simulink model "torqueBalancingPHRIStandup"  (Simulink 9.1)
settings: Solver=FixedStepDiscrete  StartTime=0.0  StopTime="Config.SIMULATION_TIME "  FixedStep=Config.Ts  RelTol=1e-3  EnableMultiTasking=on
StopFcn:
  | cd(fileparts(which(bdroot)));
  | stopTorqueBalancingPHRIStandup;
undefined symbols (not defined in the file or in its folder): ASSISTANT_DOF_FOR_SIMULINK, bVectorConstraintsFeet, bVectorConstraintsLegs, Config, ConstraintsMatrixFeet, ConstraintsMatrixLegs, Gain, Reg, ROBOT_DOF, ROBOT_DOF_FOR_SIMULINK, Sat, Sm
libraries: WBToolboxLibrary x154, simulink x4
(part 1 of 4)
settings Model: SuppressorTable=22 serialization::archive 11 0 6 0 0 0 1 0  Creator=daniele  LastModifiedBy=yeshi  NumberOfSteps=100
settings DataIOCC: LimitDataPoints=on
settings OptimizationCC: ExpressionDepthLimit=2147483647
settings DebuggingCC: SolverPrmCheckMsg=warning  FcnCallInpInsideContextMsg=warning  AllowSymbolicDim=off  StateNameClashWarn=warning
settings SFSimCC: SimParseCustomCode=off
settings GRTTargetCC: GeneratePreprocessorConditionals=Disable all

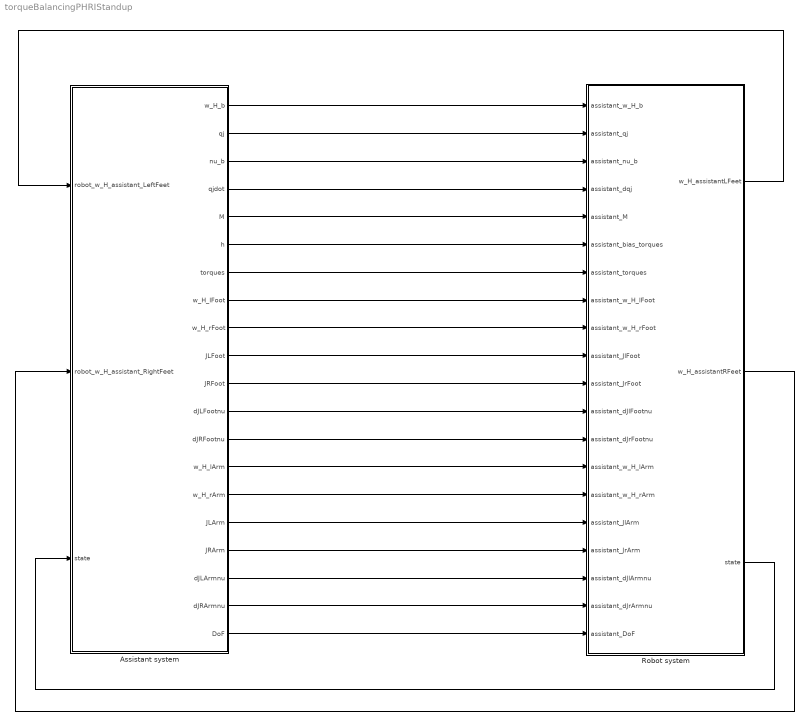
== system torqueBalancingPHRIStandup ==
  Assistant system : Subsystem
  Robot system : Subsystem
  wires:
  Assistant system/1(w_H_b) -> Robot system/1("assistant_w_H_b ")
  Assistant system/2(qj) -> Robot system/2("assistant_qj ")
  Assistant system/3(nu_b) -> Robot system/3(assistant_nu_b)
  Assistant system/4(qjdot) -> Robot system/4(assistant_dqj)
  Assistant system/5(M) -> Robot system/5(assistant_M)
  Assistant system/6(h) -> Robot system/6(assistant_bias_torques)
  Assistant system/7(torques) -> Robot system/7(assistant_torques)
  Assistant system/8(w_H_lFoot) -> Robot system/8(assistant_w_H_lFoot)
  Assistant system/9(w_H_rFoot) -> Robot system/9(assistant_w_H_rFoot)
  Assistant system/10(JLFoot) -> Robot system/10(assistant_JlFoot)
  Assistant system/11(JRFoot) -> Robot system/11(assistant_JrFoot)
  Assistant system/12(dJLFootnu) -> Robot system/12(assistant_dJlFootnu)
  Assistant system/13(dJRFootnu) -> Robot system/13(assistant_dJrFootnu)
  Assistant system/14(w_H_lArm) -> Robot system/14(assistant_w_H_lArm)
  Assistant system/15(w_H_rArm) -> Robot system/15(assistant_w_H_rArm)
  Assistant system/16(JLArm) -> Robot system/16(assistant_JlArm)
  Assistant system/17(JRArm) -> Robot system/17(assistant_JrArm)
  Assistant system/18(dJLArmnu) -> Robot system/18(assistant_dJlArmnu)
  Assistant system/19(dJRArmnu) -> Robot system/19(assistant_dJrArmnu)
  Assistant system/20(DoF) -> Robot system/20(assistant_DoF)
  Robot system/1(w_H_assistantLFeet) -> Assistant system/1(robot_w_H_assistant_LeftFeet)
  Robot system/2(w_H_assistantRFeet) -> Assistant system/2(robot_w_H_assistant_RightFeet)
  Robot system/3(state) -> Assistant system/3("state ")

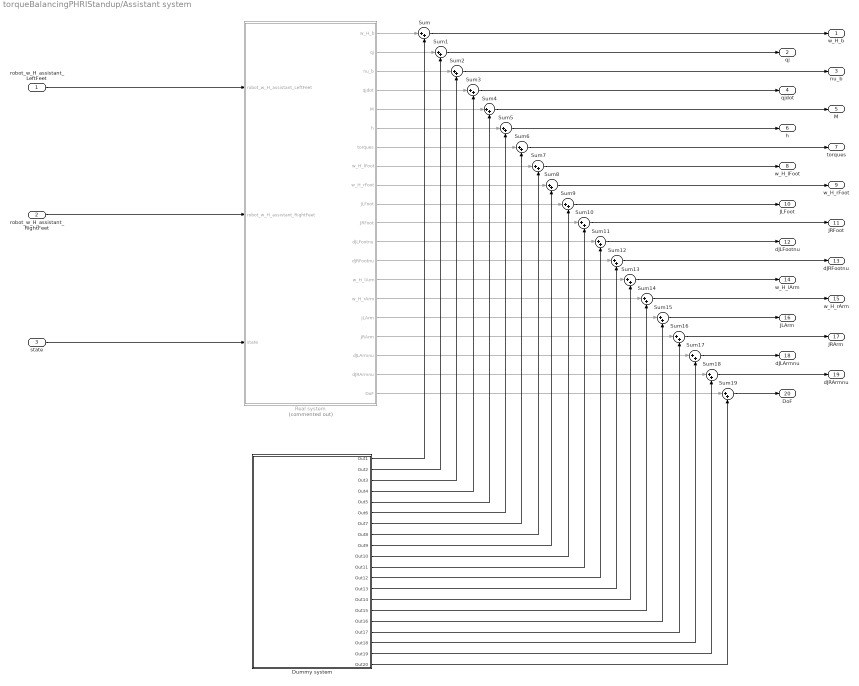
== system torqueBalancingPHRIStandup/Assistant system ==
  robot_w_H_assistant_LeftFeet : Inport
  robot_w_H_assistant_RightFeet : Inport  Port=2
  "state " : Inport  Port=3
  Dummy system : Subsystem
  Real system : Subsystem  Commented=on
  Sum{,1..19} (20 alike) : Sum  Inputs=|++
  w_H_b : Outport
  qj : Outport  Port=2
  nu_b : Outport  Port=3
  qjdot : Outport  Port=4
  M : Outport  Port=5
  h : Outport  Port=6
  torques : Outport  Port=7
  w_H_lFoot : Outport  Port=8
  w_H_rFoot : Outport  Port=9
  JLFoot : Outport  Port=10
  JRFoot : Outport  Port=11
  dJLFootnu : Outport  Port=12
  dJRFootnu : Outport  Port=13
  w_H_lArm : Outport  Port=14
  w_H_rArm : Outport  Port=15
  JLArm : Outport  Port=16
  JRArm : Outport  Port=17
  dJLArmnu : Outport  Port=18
  dJRArmnu : Outport  Port=19
  DoF : Outport  Port=20
  wires:
  robot_w_H_assistant_LeftFeet/1 -> Real system/1(robot_w_H_assistant_LeftFeet)
  robot_w_H_assistant_RightFeet/1 -> Real system/2(robot_w_H_assistant_RightFeet)
  "state "/1 -> Real system/3("state ")
  Sum/1 -> w_H_b/1
  Real system/1(w_H_b) -> Sum/1
  Real system/2(qj) -> Sum1/1
  Sum1/1 -> qj/1
  Real system/3(nu_b) -> Sum2/1
  Sum2/1 -> nu_b/1
  Real system/4(qjdot) -> Sum3/1
  Sum3/1 -> qjdot/1
  Real system/5(M) -> Sum4/1
  Sum4/1 -> M/1
  Real system/6(h) -> Sum5/1
  Sum5/1 -> h/1
  Real system/7(torques) -> Sum6/1
  Sum6/1 -> torques/1
  Real system/8(w_H_lFoot) -> Sum7/1
  Sum7/1 -> w_H_lFoot/1
  Real system/9(w_H_rFoot) -> Sum8/1
  Sum8/1 -> w_H_rFoot/1
  Real system/10(JLFoot) -> Sum9/1
  Sum9/1 -> JLFoot/1
  Real system/11(JRFoot) -> Sum10/1
  Sum10/1 -> JRFoot/1
  Real system/12(dJLFootnu) -> Sum11/1
  Sum11/1 -> dJLFootnu/1
  Real system/13(dJRFootnu) -> Sum12/1
  Sum12/1 -> dJRFootnu/1
  Real system/14(w_H_lArm) -> Sum13/1
  Sum13/1 -> w_H_lArm/1
  Real system/15(w_H_rArm) -> Sum14/1
  Sum14/1 -> w_H_rArm/1
  Real system/16(JLArm) -> Sum15/1
  Sum15/1 -> JLArm/1
  Real system/17(JRArm) -> Sum16/1
  Sum16/1 -> JRArm/1
  Real system/18(dJLArmnu) -> Sum17/1
  Sum17/1 -> dJLArmnu/1
  Real system/19(dJRArmnu) -> Sum18/1
  Sum18/1 -> dJRArmnu/1
  Sum19/1 -> DoF/1
  Real system/20(DoF) -> Sum19/1
  Dummy system/1(Out1) -> Sum/2
  Dummy system/2(Out2) -> Sum1/2
  Dummy system/3(Out3) -> Sum2/2
  Dummy system/4(Out4) -> Sum3/2
  Dummy system/5(Out5) -> Sum4/2
  Dummy system/6(Out6) -> Sum5/2
  Dummy system/7(Out7) -> Sum6/2
  Dummy system/8(Out8) -> Sum7/2
  Dummy system/9(Out9) -> Sum8/2
  Dummy system/10(Out10) -> Sum9/2
  Dummy system/11(Out11) -> Sum10/2
  Dummy system/12(Out12) -> Sum11/2
  Dummy system/13(Out13) -> Sum12/2
  Dummy system/14(Out14) -> Sum13/2
  Dummy system/15(Out15) -> Sum14/2
  Dummy system/16(Out16) -> Sum15/2
  Dummy system/17(Out17) -> Sum16/2
  Dummy system/18(Out18) -> Sum17/2
  Dummy system/19(Out19) -> Sum18/2
  Dummy system/20(Out20) -> Sum19/2

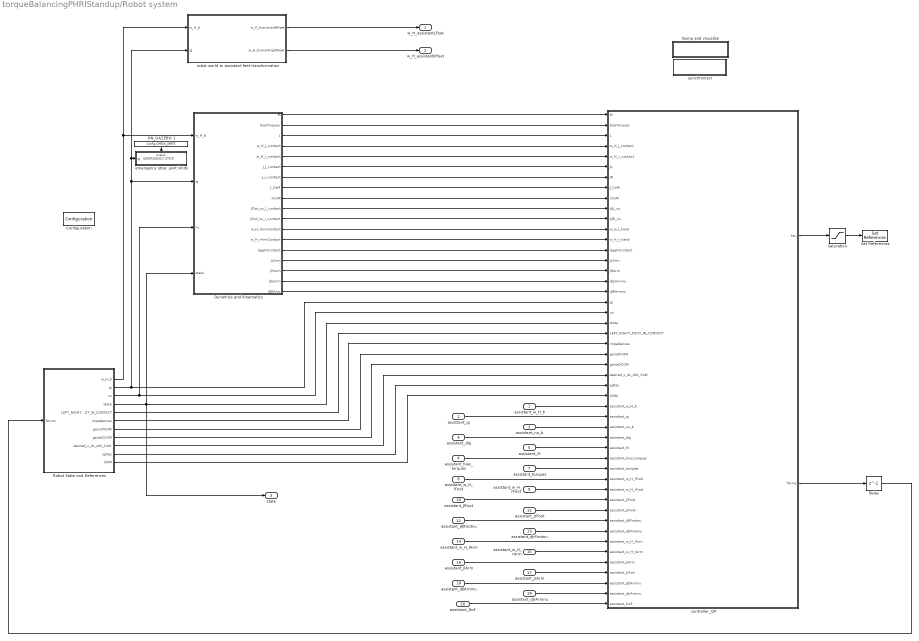
== system torqueBalancingPHRIStandup/Robot system ==
  "assistant_w_H_b " : Inport
  "assistant_qj " : Inport  Port=2
  assistant_nu_b : Inport  Port=3
  assistant_dqj : Inport  Port=4
  assistant_M : Inport  Port=5
  assistant_bias_torques : Inport  Port=6
  assistant_torques : Inport  Port=7
  assistant_w_H_lFoot : Inport  Port=8
  assistant_w_H_rFoot : Inport  Port=9
  assistant_JlFoot : Inport  Port=10
  assistant_JrFoot : Inport  Port=11
  assistant_dJlFootnu : Inport  Port=12
  assistant_dJrFootnu : Inport  Port=13
  assistant_w_H_lArm : Inport  Port=14
  assistant_w_H_rArm : Inport  Port=15
  assistant_JlArm : Inport  Port=16
  assistant_JrArm : Inport  Port=17
  assistant_dJlArmnu : Inport  Port=18
  assistant_dJrArmnu : Inport  Port=19
  assistant_DoF : Inport  Port=20
  Configuration : WBToolboxLibrary/Utilities/Configuration  ConfigSource=Workspace  ConfigObject='WBTConfigRobot'
      settings: SourceProductName=Whole Body Toolbox
  Delay : Delay  DelayLength=1
  Dump and visualize : Subsystem
      mask Display: disp('VISUALIZER')
  Dynamics and Kinematics : Subsystem
  ON_GAZEBO 1 : Constant  Value=Config.CHECK_LIMITS
  Robot State and References : Subsystem  Priority=-10
  Saturation : Saturate  UpperLimit=Sat.torque  LowerLimit=-Sat.torque
  Set References : WBToolboxLibrary/wholeBodyActuators/Set References  controlType=Torque  refSpeed=50  refAcceleration=1000000*(pi/180)
      settings: SourceProductName=Whole Body Toolbox
  controller_QP : Subsystem
  emergency stop: joint limits : Subsystem
  robot world to assistant feet transformation : Subsystem
  synchronizer : Subsystem
      mask Display: disp('SYNCHRONIZER')
  w_H_assistantLFeet : Outport
  w_H_assistantRFeet : Outport  Port=2
  state : Outport  Port=3
  wires:
  Dynamics and Kinematics/9(xCoM) -> controller_QP/9(xCoM)
  Saturation/1 -> Set References/1
  Robot State and References/6(impedances) -> controller_QP/23(impedances)
  Robot State and References/7(gainsPCOM) -> controller_QP/24(gainsPCOM)
  Dynamics and Kinematics/10(JDot_nu_l_contact) -> controller_QP/10(dJL_nu)
  Robot State and References/5(LEFT_RIGHT_FOOT_IN_CONTACT) -> controller_QP/22(LEFT_RIGHT_FOOT_IN_CONTACT)
  Dynamics and Kinematics/2(biasTorques) -> controller_QP/2(biasTorques)
  ON_GAZEBO 1/1 -> emergency stop: joint limits/Enable
  Dynamics and Kinematics/6(J_l_contact) -> controller_QP/6(JL)
  Dynamics and Kinematics/14(legsInContact) -> controller_QP/14(legsInContact)
  Dynamics and Kinematics/8(J_CoM) -> controller_QP/8(J_CoM)
  Robot State and References/4(state) -> state/1, Dynamics and Kinematics/4("state "), controller_QP/21(state)
  Dynamics and Kinematics/4(w_H_l_contact) -> controller_QP/4(w_H_l_contact)
  Robot State and References/2(qj) -> robot world to assistant feet transformation/2(qj), emergency stop: joint limits/1(qj   EMERGENCY STOP), Dynamics and Kinematics/2(qj), controller_QP/19(qj)
  Dynamics and Kinematics/11(JDot_nu_r_contact) -> controller_QP/11(dJR_nu)
  Robot State and References/10(qjDes) -> controller_QP/27(qjDes)
  Robot State and References/9(desired_x_dx_ddx_CoM) -> controller_QP/26(desired_x_dx_ddx_CoM)
  Dynamics and Kinematics/1(M) -> controller_QP/1(M)
  Dynamics and Kinematics/5(w_H_r_contact) -> controller_QP/5(w_H_r_contact)
  Robot State and References/8(gainsDCOM) -> controller_QP/25(gainsDCOM)
  Robot State and References/1(w_H_b) -> robot world to assistant feet transformation/1(w_H_b), Dynamics and Kinematics/1(w_H_b)
  Robot State and References/3(nu) -> Dynamics and Kinematics/3(nu), controller_QP/20(nu)
  controller_QP/1("tau ") -> Saturation/1
  Dynamics and Kinematics/7(J_r_contact) -> controller_QP/7(JR)
  Dynamics and Kinematics/3(L) -> controller_QP/3("L ")
  robot world to assistant feet transformation/2(w_H_humanRightFeet) -> w_H_assistantRFeet/1
  robot world to assistant feet transformation/1(w_H_humanLeftFeet) -> w_H_assistantLFeet/1
  "assistant_w_H_b "/1 -> controller_QP/29("assistant_w_H_b ")
  "assistant_qj "/1 -> controller_QP/30("assistant_qj ")
  assistant_nu_b/1 -> controller_QP/31(assistant_nu_b)
  assistant_dqj/1 -> controller_QP/32(assistant_dqj)
  assistant_M/1 -> controller_QP/33(assistant_M)
  assistant_bias_torques/1 -> controller_QP/34(assistant_bias_torques)
  assistant_torques/1 -> controller_QP/35(assistant_torques)
  assistant_w_H_lFoot/1 -> controller_QP/36(assistant_w_H_lFoot)
  assistant_w_H_rFoot/1 -> controller_QP/37(assistant_w_H_rFoot)
  assistant_JlFoot/1 -> controller_QP/38(assistant_JlFoot)
  assistant_JrFoot/1 -> controller_QP/39(assistant_JrFoot)
  assistant_dJlFootnu/1 -> controller_QP/40(assistant_dJlFootnu)
  assistant_dJrFootnu/1 -> controller_QP/41(assistant_dJrFootnu)
  assistant_w_H_lArm/1 -> controller_QP/42(assistant_w_H_lArm)
  assistant_w_H_rArm/1 -> controller_QP/43(assistant_w_H_rArm)
  assistant_JlArm/1 -> controller_QP/44(assistant_JlArm)
  assistant_JrArm/1 -> controller_QP/45(assistant_JrArm)
  assistant_dJlArmnu/1 -> controller_QP/46(assistant_dJlArmnu)
  assistant_dJrArmnu/1 -> controller_QP/47(assistant_dJrArmnu)
  assistant_DoF/1 -> controller_QP/48(assistant_DoF)
  Dynamics and Kinematics/12(w_H_lArmContact) -> controller_QP/12(w_H_l_hand)
  Dynamics and Kinematics/13(w_H_rArmContact) -> controller_QP/13(w_H_r_hand)
  Dynamics and Kinematics/15(JLArm) -> controller_QP/15(JLArm)
  Dynamics and Kinematics/16(JRArm) -> controller_QP/16(JRArm)
  Dynamics and Kinematics/17(dJLArm) -> controller_QP/17(dJLArmnu)
  Dynamics and Kinematics/18(dJRArm) -> controller_QP/18(dJRArmnu)
  controller_QP/2(fArms) -> Delay/1
  Delay/1 -> Robot State and References/1(fArms)
  Robot State and References/11(CMM) -> controller_QP/28(CMM)

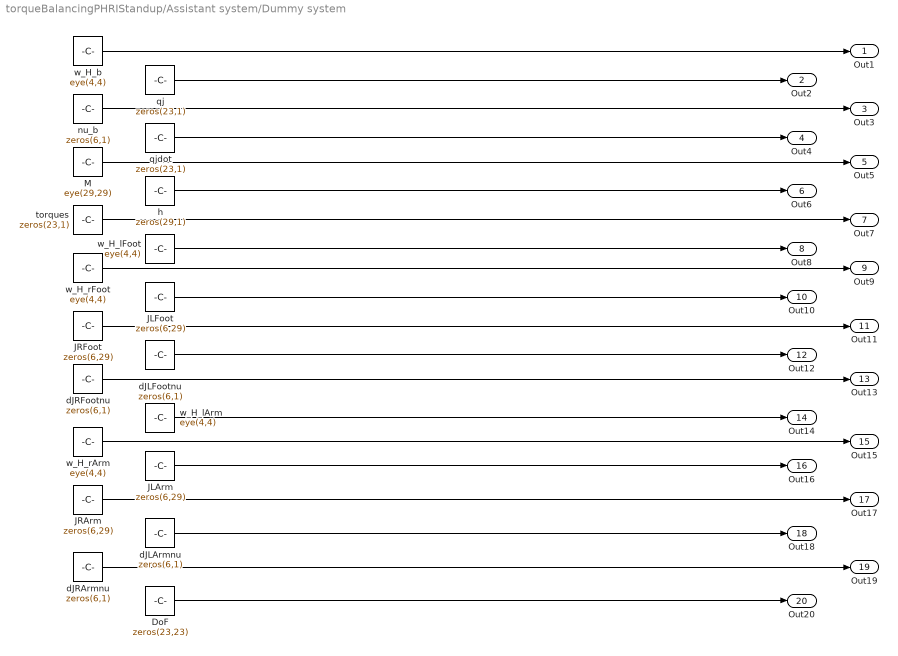
== system torqueBalancingPHRIStandup/Assistant system/Dummy system ==
  DoF : Constant  Value=zeros(23,23)
  JLArm : Constant  Value=zeros(6,29)
  "JLFoot " : Constant  Value=zeros(6,29)
  JRArm : Constant  Value=zeros(6,29)
  JRFoot : Constant  Value=zeros(6,29)
  M : Constant  Value=eye(29,29)
  dJLArmnu : Constant  Value=zeros(6,1)
  dJLFootnu : Constant  Value=zeros(6,1)
  dJRArmnu : Constant  Value=zeros(6,1)
  dJRFootnu : Constant  Value=zeros(6,1)
  "h " : Constant  Value=zeros(29,1)
  nu_b : Constant  Value=zeros(6,1)
  qj : Constant  Value=zeros(23,1)
  qjdot : Constant  Value=zeros(23,1)
  torques : Constant  Value=zeros(23,1)
  w_H_b : Constant  Value=eye(4,4)
  "w_H_lArm " : Constant  Value=eye(4,4)
  w_H_lFoot : Constant  Value=eye(4,4)
  "w_H_rArm " : Constant  Value=eye(4,4)
  "w_H_rFoot " : Constant  Value=eye(4,4)
  Out1 : Outport
  Out2 : Outport  Port=2
  Out3 : Outport  Port=3
  Out4 : Outport  Port=4
  Out5 : Outport  Port=5
  Out6 : Outport  Port=6
  Out7 : Outport  Port=7
  Out8 : Outport  Port=8
  Out9 : Outport  Port=9
  Out10 : Outport  Port=10
  Out11 : Outport  Port=11
  Out12 : Outport  Port=12
  Out13 : Outport  Port=13
  Out14 : Outport  Port=14
  Out15 : Outport  Port=15
  Out16 : Outport  Port=16
  Out17 : Outport  Port=17
  Out18 : Outport  Port=18
  Out19 : Outport  Port=19
  Out20 : Outport  Port=20
  wires:
  nu_b/1 -> Out3/1
  DoF/1 -> Out20/1
  JRArm/1 -> Out17/1
  "w_H_lArm "/1 -> Out14/1
  "w_H_rArm "/1 -> Out15/1
  dJRArmnu/1 -> Out19/1
  w_H_lFoot/1 -> Out8/1
  "JLFoot "/1 -> Out10/1
  torques/1 -> Out7/1
  qjdot/1 -> Out4/1
  w_H_b/1 -> Out1/1
  dJRFootnu/1 -> Out13/1
  dJLArmnu/1 -> Out18/1
  qj/1 -> Out2/1
  "h "/1 -> Out6/1
  dJLFootnu/1 -> Out12/1
  "w_H_rFoot "/1 -> Out9/1
  JRFoot/1 -> Out11/1
  JLArm/1 -> Out16/1
  M/1 -> Out5/1

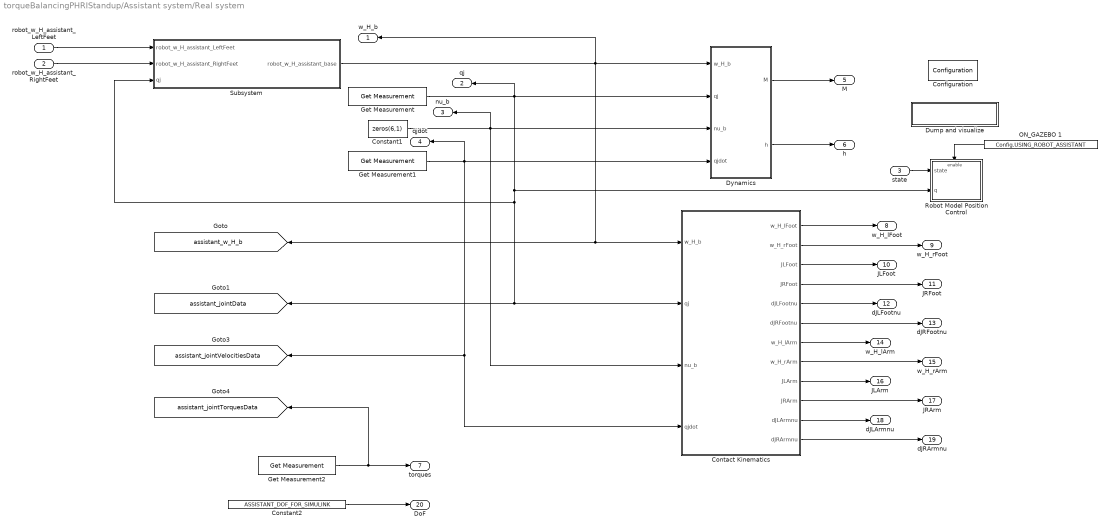
== system torqueBalancingPHRIStandup/Assistant system/Real system ==
  robot_w_H_assistant_LeftFeet : Inport
  robot_w_H_assistant_RightFeet : Inport  Port=2
  "state " : Inport  Port=3
  Configuration : WBToolboxLibrary/Utilities/Configuration  ConfigSource=Workspace  ConfigObject='ASSISTANT_WBTConfigRobot'
      settings: SourceProductName=Whole Body Toolbox
  Constant1 : Constant  Value=zeros(6,1)
  Constant2 : Constant  Value=ASSISTANT_DOF_FOR_SIMULINK
  Contact Kinematics : Subsystem
  Dump and visualize : Subsystem
      mask Display: disp('VISUALIZER')
  Dynamics : Subsystem
  Get Measurement : WBToolboxLibrary/wholeBodyStates/Get Measurement  measuredType=Joints Position
      settings: SourceProductName=Whole Body Toolbox
  Get Measurement1 : WBToolboxLibrary/wholeBodyStates/Get Measurement  measuredType=Joints Velocity
      settings: SourceProductName=Whole Body Toolbox
  Get Measurement2 : WBToolboxLibrary/wholeBodyStates/Get Measurement  measuredType=Joints Torque
      settings: SourceProductName=Whole Body Toolbox
  ON_GAZEBO 1 : Constant  Value=Config.USING_ROBOT_ASSISTANT
  Robot Model Position Control : Subsystem
  Subsystem : Subsystem
  w_H_b : Outport
  qj : Outport  Port=2
  nu_b : Outport  Port=3
  qjdot : Outport  Port=4
  M : Outport  Port=5
  h : Outport  Port=6
  torques : Outport  Port=7
  w_H_lFoot : Outport  Port=8
  w_H_rFoot : Outport  Port=9
  JLFoot : Outport  Port=10
  JRFoot : Outport  Port=11
  dJLFootnu : Outport  Port=12
  dJRFootnu : Outport  Port=13
  w_H_lArm : Outport  Port=14
  w_H_rArm : Outport  Port=15
  JLArm : Outport  Port=16
  JRArm : Outport  Port=17
  dJLArmnu : Outport  Port=18
  dJRArmnu : Outport  Port=19
  DoF : Outport  Port=20
  tag scope: assistant_jointData=global, assistant_jointTorquesData=global, assistant_jointVelocitiesData=global, assistant_w_H_b=global
  wires:
  Contact Kinematics/7(w_H_lArm) -> w_H_lArm/1
  Constant2/1 -> DoF/1
  Dynamics/1(M) -> M/1
  Dynamics/2(h) -> h/1
  Contact Kinematics/3(JLFoot) -> JLFoot/1
  robot_w_H_assistant_RightFeet/1 -> Subsystem/2(robot_w_H_assistant_RightFeet)
  Contact Kinematics/6(dJRFootnu) -> dJRFootnu/1
  Get Measurement2/1 -> torques/1, [assistant_jointTorquesData]
  Contact Kinematics/5(dJLFootnu) -> dJLFootnu/1
  robot_w_H_assistant_LeftFeet/1 -> Subsystem/1(robot_w_H_assistant_LeftFeet)
  Get Measurement1/1 -> qjdot/1, Dynamics/4(qjdot), [assistant_jointVelocitiesData], Contact Kinematics/4(qjdot)
  Contact Kinematics/12(dJRArmnu) -> dJRArmnu/1
  "state "/1 -> Robot Model Position Control/1(state)
  ON_GAZEBO 1/1 -> Robot Model Position Control/Enable
  Get Measurement/1 -> qj/1, [assistant_jointData], Contact Kinematics/2(qj), Subsystem/3(qj), Robot Model Position Control/2(q), Dynamics/2(qj)
  Subsystem/1(robot_w_H_assistant_base) -> w_H_b/1, Contact Kinematics/1(w_H_b), [assistant_w_H_b], Dynamics/1(w_H_b)
  Contact Kinematics/8(w_H_rArm) -> w_H_rArm/1
  Constant1/1 -> nu_b/1, Contact Kinematics/3(nu_b), Dynamics/3(nu_b)
  Contact Kinematics/10(JRArm) -> JRArm/1
  Contact Kinematics/4(JRFoot) -> JRFoot/1
  Contact Kinematics/1(w_H_lFoot) -> w_H_lFoot/1
  Contact Kinematics/9(JLArm) -> JLArm/1
  Contact Kinematics/11(dJLArmnu) -> dJLArmnu/1
  Contact Kinematics/2(w_H_rFoot) -> w_H_rFoot/1

== system torqueBalancingPHRIStandup/Robot system/Dump and visualize ==
  Human assistance : Subsystem
  Logical Operator2 : Logic  Operator=OR  AllPortsSameDT=off  OutDataTypeStr=boolean
  ON_GAZEBO 1 : Constant  Value=Config.SCOPES_ALL
  ON_GAZEBO 2 : Constant  Value=Config.SCOPES_MAIN
  Robot data1 : Subsystem
  wires:
  [alpha] -> Human assistance/2(alpha)
  [fArms] -> Human assistance/3(fArms)
  [phri_assistant_feet_wrench] -> Human assistance/4(phri_assistant_feet_wrench)
  [phri_robot_feet_wrench] -> Human assistance/5(phri_robot_feet_wrench)
  [f_noQP] -> Robot data1/8(fDesNoQP)
  ON_GAZEBO 2/1 -> Logical Operator2/2
  [CoM_error] -> Robot data1/5(CoM_Error)
  [state] -> Human assistance/1(state), Robot data1/3(state)
  [qj_des] -> Robot data1/4(qj_des)
  [CoM_des] -> Robot data1/7(CoM_des)
  [w_H_b] -> Robot data1/2(w_H_b)
  Logical Operator2/1 -> Robot data1/Enable
  ON_GAZEBO 1/1 -> Logical Operator2/1
  [tau_des] -> Robot data1/1(tau_des)
  [f_QP] -> Robot data1/6(fDesQP)

== system torqueBalancingPHRIStandup/Robot system/Dynamics and Kinematics ==
  w_H_b : Inport
  qj : Inport  Port=2
  nu : Inport  Port=3
  "state " : Inport  Port=4
  Dynamics : Subsystem
  Kinematics : Subsystem
  M : Outport
  biasTorques : Outport  Port=2
  L : Outport  Port=3
  w_H_l_contact : Outport  Port=4
  w_H_r_contact : Outport  Port=5
  J_l_contact : Outport  Port=6
  J_r_contact : Outport  Port=7
  J_CoM : Outport  Port=8
  xCoM : Outport  Port=9
  JDot_nu_l_contact : Outport  Port=10
  JDot_nu_r_contact : Outport  Port=11
  w_H_lArmContact : Outport  Port=12
  w_H_rArmContact : Outport  Port=13
  legsInContact : Outport  Port=14
  JLArm : Outport  Port=15
  JRArm : Outport  Port=16
  dJLArm : Outport  Port=17
  dJRArm : Outport  Port=18
  wires:
  w_H_b/1 -> Kinematics/3(w_H_b), Dynamics/1(w_H_b)
  qj/1 -> Dynamics/2(qj), Kinematics/2(qj)
  nu/1 -> Dynamics/3(nu), Kinematics/1(nu)
  Dynamics/1(M(q)) -> M/1
  Dynamics/2(biasTorques) -> biasTorques/1
  Dynamics/3(L(q,dq)) -> L/1
  Kinematics/5(J_CoM) -> J_CoM/1
  Kinematics/6(xCoM) -> xCoM/1
  Kinematics/1(w_H_l_contact) -> w_H_l_contact/1
  Kinematics/2(w_H_r_contact) -> w_H_r_contact/1
  Kinematics/7(JDot_nu_l_contact) -> JDot_nu_l_contact/1
  Kinematics/8(JDot_nu_r_contact) -> JDot_nu_r_contact/1
  Kinematics/3(J_l_contact) -> J_l_contact/1
  Kinematics/4(J_r_contact) -> J_r_contact/1
  Kinematics/9(legsInContact) -> legsInContact/1
  "state "/1 -> Kinematics/4("state ")
  Kinematics/12(JLArm) -> JLArm/1
  Kinematics/11(w_H_rArmContact) -> w_H_rArmContact/1
  Kinematics/13(JRArm) -> JRArm/1
  Kinematics/15(JDot_nu_rArm_contact) -> dJRArm/1
  Kinematics/14(JDot_nu_lArm_contact) -> dJLArm/1
  Kinematics/10(w_H_lArmContact) -> w_H_lArmContact/1

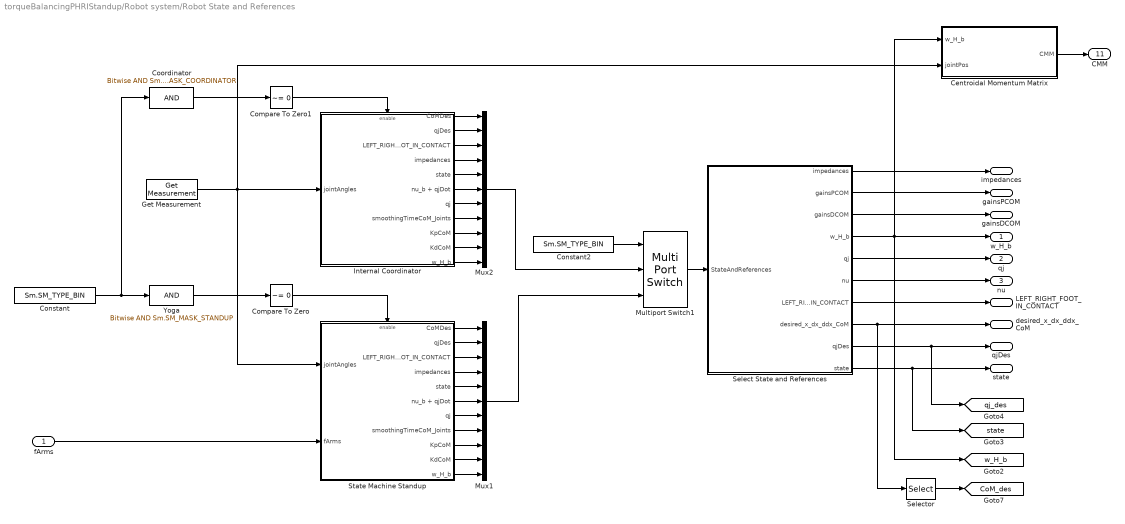
== system torqueBalancingPHRIStandup/Robot system/Robot State and References ==
  fArms : Inport
  "Centroidal Momentum Matrix " : Subsystem
  Compare To Zero : simulink/Logic and Bit Operations/Compare To Zero  relop=~=  OutDataTypeStr=boolean
  Compare To Zero1 : simulink/Logic and Bit Operations/Compare To Zero  relop=~=  OutDataTypeStr=boolean
  Constant : Constant  Priority=-10  Value=Sm.SM_TYPE_BIN  OutDataTypeStr=uint8
  Constant2 : Constant  Priority=-10  Value=Sm.SM_TYPE_BIN  OutDataTypeStr=uint8
  Coordinator : simulink/Logic and Bit Operations/Bitwise Operator  logicop=AND  UseBitMask=on  BitMask=Sm.SM_MASK_COORDINATOR  BitMaskRealWorld=Stored Integer
  Get Measurement : WBToolboxLibrary/wholeBodyStates/Get Measurement  measuredType=Joints Position
      settings: SourceProductName=Whole Body Toolbox
  Internal Coordinator : Subsystem
  Multiport Switch1 : MultiPortSwitch  DataPortOrder=Specify indices  DataPortIndices={1, 2}
  Mux1 : Mux  Inputs=11
  Mux2 : Mux  Inputs=11
  Select State and References : Subsystem
  Selector : Selector  NumberOfDimensions=2  InputPortWidth=3  IndexOptions=Index vector (dialog),Index vector (dialog)  Indices=[1 2 3],[1]  OutputSizes=1,1
  State Machine Standup : Subsystem  Priority=-100
  Yoga : simulink/Logic and Bit Operations/Bitwise Operator  logicop=AND  UseBitMask=on  BitMask=Sm.SM_MASK_STANDUP  BitMaskRealWorld=Stored Integer
  w_H_b : Outport
  qj : Outport  Port=2
  nu : Outport  Port=3
  state : Outport  Port=4
  LEFT_RIGHT_FOOT_IN_CONTACT : Outport  Port=5
  impedances : Outport  Port=6
  gainsPCOM : Outport  Port=7
  gainsDCOM : Outport  Port=8
  desired_x_dx_ddx_CoM : Outport  Port=9
  qjDes : Outport  Port=10
  CMM : Outport  Port=11
  tag scope: CoM_des=global, qj_des=global, state=global, w_H_b=global
  wires:
  Constant/1 -> Yoga/1, Coordinator/1
  State Machine Standup/3(LEFT_RIGHT_FOOT_IN_CONTACT) -> Mux1/3
  State Machine Standup/2(qjDes) -> Mux1/2
  State Machine Standup/1(CoMDes) -> Mux1/1
  Internal Coordinator/1(CoMDes) -> Mux2/1
  Internal Coordinator/2(qjDes) -> Mux2/2
  Internal Coordinator/3(LEFT_RIGHT_FOOT_IN_CONTACT) -> Mux2/3
  State Machine Standup/4(impedances) -> Mux1/4
  Internal Coordinator/4(impedances) -> Mux2/4
  State Machine Standup/5(state) -> Mux1/5
  Internal Coordinator/5(state) -> Mux2/5
  Internal Coordinator/6(nu_b + qjDot) -> Mux2/6
  Internal Coordinator/7(qj) -> Mux2/7
  State Machine Standup/6(nu_b + qjDot) -> Mux1/6
  State Machine Standup/7(qj) -> Mux1/7
  Coordinator/1 -> Compare To Zero1/1
  Yoga/1 -> Compare To Zero/1
  Compare To Zero/1 -> State Machine Standup/Enable
  Compare To Zero1/1 -> Internal Coordinator/Enable
  Internal Coordinator/8(smoothingTimeCoM_Joints) -> Mux2/8
  State Machine Standup/8(smoothingTimeCoM_Joints) -> Mux1/8
  State Machine Standup/9(KpCoM) -> Mux1/9
  State Machine Standup/10(KdCoM) -> Mux1/10
  Internal Coordinator/9(KpCoM) -> Mux2/9
  Internal Coordinator/10(KdCoM) -> Mux2/10
  Constant2/1 -> Multiport Switch1/1
  Get Measurement/1 -> "Centroidal Momentum Matrix "/2(jointPos), Internal Coordinator/1(jointAngles), State Machine Standup/1(jointAngles)
  State Machine Standup/11(w_H_b) -> Mux1/11
  Internal Coordinator/11(w_H_b) -> Mux2/11
  Mux2/1 -> Multiport Switch1/2
  Multiport Switch1/1 -> Select State and References/1(StateAndReferences)
  Select State and References/1(impedances) -> impedances/1
  Select State and References/2(gainsPCOM) -> gainsPCOM/1
  Select State and References/3(gainsDCOM) -> gainsDCOM/1
  Select State and References/4(w_H_b) -> "Centroidal Momentum Matrix "/1(w_H_b), w_H_b/1, [w_H_b]
  Select State and References/5(qj) -> qj/1
  Select State and References/6(nu) -> nu/1
  Select State and References/7(LEFT_RIGHT_FOOT_IN_CONTACT) -> LEFT_RIGHT_FOOT_IN_CONTACT/1
  Select State and References/8(desired_x_dx_ddx_CoM) -> desired_x_dx_ddx_CoM/1, Selector/1
  Select State and References/9(qjDes) -> qjDes/1, [qj_des]
  Select State and References/10(state) -> state/1, [state]
  Selector/1 -> [CoM_des]
  Mux1/1 -> Multiport Switch1/3
  fArms/1 -> State Machine Standup/2(fArms)
  "Centroidal Momentum Matrix "/1(CMM) -> CMM/1

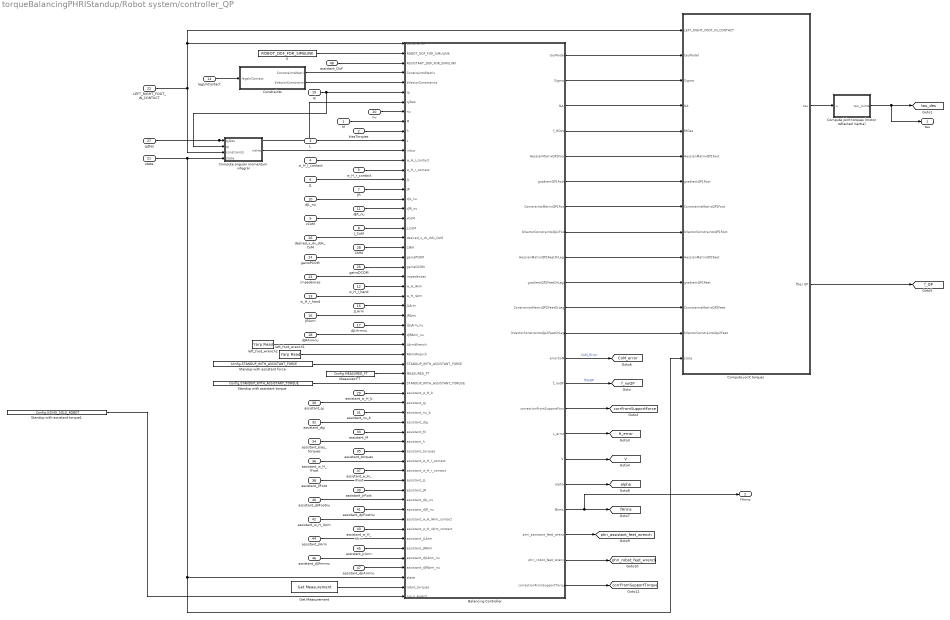
== system torqueBalancingPHRIStandup/Robot system/controller_QP ==
  M : Inport
  biasTorques : Inport  Port=2
  "L " : Inport  Port=3
  w_H_l_contact : Inport  Port=4
  w_H_r_contact : Inport  Port=5
  JL : Inport  Port=6
  JR : Inport  Port=7
  J_CoM : Inport  Port=8
  xCoM : Inport  Port=9
  dJL_nu : Inport  Port=10
  dJR_nu : Inport  Port=11
  w_H_l_hand : Inport  Port=12
  w_H_r_hand : Inport  Port=13
  legsInContact : Inport  Port=14
  JLArm : Inport  Port=15
  JRArm : Inport  Port=16
  dJLArmnu : Inport  Port=17
  dJRArmnu : Inport  Port=18
  qj : Inport  Port=19
  nu : Inport  Port=20
  state : Inport  Port=21
  LEFT_RIGHT_FOOT_IN_CONTACT : Inport  Port=22
  impedances : Inport  Port=23
  gainsPCOM : Inport  Port=24
  gainsDCOM : Inport  Port=25
  desired_x_dx_ddx_CoM : Inport  Port=26
  qjDes : Inport  Port=27
  CMM : Inport  Port=28
  "assistant_w_H_b " : Inport  Port=29
  "assistant_qj " : Inport  Port=30
  assistant_nu_b : Inport  Port=31
  assistant_dqj : Inport  Port=32
  assistant_M : Inport  Port=33
  assistant_bias_torques : Inport  Port=34
  assistant_torques : Inport  Port=35
  assistant_w_H_lFoot : Inport  Port=36
  assistant_w_H_rFoot : Inport  Port=37
  assistant_JlFoot : Inport  Port=38
  assistant_JrFoot : Inport  Port=39
  assistant_dJlFootnu : Inport  Port=40
  assistant_dJrFootnu : Inport  Port=41
  assistant_w_H_lArm : Inport  Port=42
  assistant_w_H_rArm : Inport  Port=43
  assistant_JlArm : Inport  Port=44
  assistant_JrArm : Inport  Port=45
  assistant_dJlArmnu : Inport  Port=46
  assistant_dJrArmnu : Inport  Port=47
  assistant_DoF : Inport  Port=48
  "    5" : Constant  Value=ROBOT_DOF_FOR_SIMULINK
  "Balancing Controller " : MATLAB Function  TreatAsAtomicUnit=on
  Compute angular momentum integral : Subsystem
  Compute joint torques : Subsystem
  Compute joint torques (motor reflected inertia) : Subsystem
  Constraints : Subsystem
  Get Measurement : WBToolboxLibrary/wholeBodyStates/Get Measurement  measuredType=Joints Torque
      settings: SourceProductName=Whole Body Toolbox
  Measured FT : Constant  Value=Config.MEASURED_FT
  Standup with assistant force : Constant  Value=Config.STANDUP_WITH_ASSISTANT_FORCE
  Standup with assistant torque : Constant  Value=Config.STANDUP_WITH_ASSISTANT_TORQUE
  Standup with assistant torque1 : Constant  Value=Config.USING_SOLO_ROBOT
  left_foot_wrench1 : WBToolboxLibrary/Utilities/Yarp Read  portName=Ports.RIGHT_ARM  signalSize=6  timeout=0.5  blocking=off  timestamp=off  autoconnect=on  errorOnConnection=on
      settings: SourceProductName=Whole Body Toolbox
  left_foot_wrench2 : WBToolboxLibrary/Utilities/Yarp Read  portName=Ports.LEFT_ARM  signalSize=6  timeout=0.5  blocking=off  timestamp=off  autoconnect=on  errorOnConnection=on
      settings: SourceProductName=Whole Body Toolbox
  "tau " : Outport
  fArms : Outport  Port=2
  tag scope: CoM_error=global, H_error=global, V=global, alpha=global, corrFromSupportForce=global, corrFromSupportTorque=global, fArms=global, f_QP=global, f_noQP=global, phri_assistant_feet_wrench=global, phri_robot_feet_wrench=global, tau_des=global
  wires:
  LEFT_RIGHT_FOOT_IN_CONTACT/1 -> Compute joint torques/1(LEFT_RIGHT_FOOT_IN_CONTACT), "Balancing Controller "/1(constraints), Compute angular momentum integral/3(constraints)
  qj/1 -> "Balancing Controller "/6(qj), Compute angular momentum integral/2(qj)
  qjDes/1 -> "Balancing Controller "/7(qjDes), Compute angular momentum integral/1(qjDes)
  M/1 -> "Balancing Controller "/9(M)
  biasTorques/1 -> "Balancing Controller "/10(h)
  desired_x_dx_ddx_CoM/1 -> "Balancing Controller "/21(desired_x_dx_ddx_CoM)
  impedances/1 -> "Balancing Controller "/25(impedances)
  "L "/1 -> "Balancing Controller "/11(L)
  "    5"/1 -> "Balancing Controller "/2(ROBOT_DOF_FOR_SIMULINK)
  Constraints/1(ConstraintsMatrix) -> "Balancing Controller "/4(ConstraintsMatrix)
  Constraints/2(bVectorConstraints) -> "Balancing Controller "/5(bVectorConstraints)
  nu/1 -> "Balancing Controller "/8(nu)
  gainsPCOM/1 -> "Balancing Controller "/23(gainsPCOM)
  gainsDCOM/1 -> "Balancing Controller "/24(gainsDCOM)
  w_H_r_contact/1 -> "Balancing Controller "/14(w_H_r_contact)
  w_H_l_contact/1 -> "Balancing Controller "/13(w_H_l_contact)
  JL/1 -> "Balancing Controller "/15(JL)
  JR/1 -> "Balancing Controller "/16(JR)
  Compute angular momentum integral/1(intHw) -> "Balancing Controller "/12(intLw)
  dJL_nu/1 -> "Balancing Controller "/17(dJL_nu)
  dJR_nu/1 -> "Balancing Controller "/18(dJR_nu)
  J_CoM/1 -> "Balancing Controller "/20(J_CoM)
  xCoM/1 -> "Balancing Controller "/19(xCoM)
  state/1 -> Compute joint torques/14(state), "Balancing Controller "/56(state), Compute angular momentum integral/4(state)
  Compute joint torques/1("tau ") -> Compute joint torques (motor reflected inertia)/1(u)
  "Balancing Controller "/1(tauModel) -> Compute joint torques/2(tauModel)
  "Balancing Controller "/2(Sigma) -> Compute joint torques/3(Sigma)
  "Balancing Controller "/3(NA) -> Compute joint torques/4(NA)
  "Balancing Controller "/4(f_HDot) -> Compute joint torques/5(fHDes)
  "Balancing Controller "/5(HessianMatrixQP1Foot) -> Compute joint torques/6(HessianMatrixQP1Foot)
  "Balancing Controller "/6(gradientQP1Foot) -> Compute joint torques/7(gradientQP1Foot)
  "Balancing Controller "/7(ConstraintsMatrixQP1Foot) -> Compute joint torques/8(ConstraintsMatrixQP1Foot)
  "Balancing Controller "/8(bVectorConstraintsQp1Foot) -> Compute joint torques/9(bVectorConstraintsQP1Foot)
  "Balancing Controller "/9(HessianMatrixQP2FeetOrLegs) -> Compute joint torques/10(HessianMatrixQP2Feet)
  "Balancing Controller "/10(gradientQP2FeetOrLegs) -> Compute joint torques/11(gradientQP2Feet)
  "Balancing Controller "/11(ConstraintsMatrixQP2FeetOrLegs) -> Compute joint torques/12(ConstraintsMatrixQP2Feet)
  "Balancing Controller "/12(bVectorConstraintsQp2FeetOrLegs) -> Compute joint torques/13(bVectorConstraintsQp2Feet)
  "Balancing Controller "/13(errorCoM) -> [CoM_error]  "CoM_Error"
  Compute joint torques/2(fDes QP) -> [f_QP]
  "Balancing Controller "/14(f_noQP) -> [f_noQP]  "fNoQP"
  Standup with assistant force/1 -> "Balancing Controller "/34(STANDUP_WITH_ASSISTANT_FORCE)
  left_foot_wrench2/1 -> "Balancing Controller "/32(LArmWrench)
  left_foot_wrench1/1 -> "Balancing Controller "/33(RArmWrench)
  w_H_l_hand/1 -> "Balancing Controller "/26(w_H_lArm)
  w_H_r_hand/1 -> "Balancing Controller "/27(w_H_rArm)
  legsInContact/1 -> Constraints/1(legsInContact)
  "Balancing Controller "/17(V) -> [V]
  "Balancing Controller "/16(L_error) -> [H_error]
  "Balancing Controller "/15(correctionFromSupportForce) -> [corrFromSupportForce]
  Compute joint torques (motor reflected inertia)/1(tau_joints) -> [tau_des], "tau "/1
  Standup with assistant torque/1 -> "Balancing Controller "/36(STANDUP_WITH_ASSISTANT_TORQUE)
  assistant_DoF/1 -> "Balancing Controller "/3(ASSISTANT_DOF_FOR_SIMULINK)
  "assistant_w_H_b "/1 -> "Balancing Controller "/37(assistant_w_H_b)
  "assistant_qj "/1 -> "Balancing Controller "/38(assistant_qj)
  assistant_nu_b/1 -> "Balancing Controller "/39(assistant_nu_b)
  assistant_dqj/1 -> "Balancing Controller "/40(assistant_dqj)
  assistant_M/1 -> "Balancing Controller "/41(assistant_M)
  assistant_bias_torques/1 -> "Balancing Controller "/42(assistant_h)
  assistant_torques/1 -> "Balancing Controller "/43(assistant_torques)
  assistant_w_H_lFoot/1 -> "Balancing Controller "/44(assistant_w_H_l_contact)
  assistant_w_H_rFoot/1 -> "Balancing Controller "/45(assistant_w_H_r_contact)
  assistant_JlFoot/1 -> "Balancing Controller "/46(assistant_JL)
  assistant_JrFoot/1 -> "Balancing Controller "/47(assistant_JR)
  assistant_dJlFootnu/1 -> "Balancing Controller "/48(assistant_dJL_nu)
  assistant_dJrFootnu/1 -> "Balancing Controller "/49(assistant_dJR_nu)
  assistant_w_H_lArm/1 -> "Balancing Controller "/50(assistant_w_H_lArm_contact)
  assistant_w_H_rArm/1 -> "Balancing Controller "/51(assistant_w_H_rArm_contact)
  assistant_JlArm/1 -> "Balancing Controller "/52(assistant_JLArm)
  assistant_JrArm/1 -> "Balancing Controller "/53(assistant_JRArm)
  assistant_dJlArmnu/1 -> "Balancing Controller "/54(assistant_dJLArm_nu)
  assistant_dJrArmnu/1 -> "Balancing Controller "/55(assistant_dJRArm_nu)
  Get Measurement/1 -> "Balancing Controller "/57(robot_torques)
  "Balancing Controller "/19(fArms) -> fArms/1, [fArms]
  "Balancing Controller "/18(alpha) -> [alpha]
  "Balancing Controller "/20(phri_assistant_feet_wrench) -> [phri_assistant_feet_wrench]
  "Balancing Controller "/21(phri_robot_feet_wrench) -> [phri_robot_feet_wrench]
  JLArm/1 -> "Balancing Controller "/28(JLArm)
  JRArm/1 -> "Balancing Controller "/29(JRArm)
  dJLArmnu/1 -> "Balancing Controller "/30(dJLArm_nu)
  dJRArmnu/1 -> "Balancing Controller "/31(dJRArm_nu)
  Measured FT/1 -> "Balancing Controller "/35(MEASURED_FT)
  CMM/1 -> "Balancing Controller "/22(CMM)
  "Balancing Controller "/22(correctionFromSupportTorque) -> [corrFromSupportTorque]
  Standup with assistant torque1/1 -> "Balancing Controller "/58(SOLO_ROBOT)

== system torqueBalancingPHRIStandup/Robot system/emergency stop: joint limits ==
  qj   EMERGENCY STOP : Inport
  Enable : EnablePort
  Assertion : Assertion
  Get Limits : WBToolboxLibrary/wholeBodyStates/Get Limits  limitsSource=ControlBoard  limitsType=Position
      settings: SourceProductName=Whole Body Toolbox
  MATLAB Function : MATLAB Function  TreatAsAtomicUnit=on
  index1 : Constant  Value=0.01  VectorParams1D=off
  wires:
  Get Limits/1 -> MATLAB Function/1(umin)
  Get Limits/2 -> MATLAB Function/2(umax)
  index1/1 -> MATLAB Function/4(tol)
  qj   EMERGENCY STOP/1 -> MATLAB Function/3(u)
  MATLAB Function/1(inRange) -> Assertion/1

== system torqueBalancingPHRIStandup/Robot system/robot world to assistant feet transformation ==
  w_H_b : Inport
  qj : Inport  Port=2
  Display{1..4} (4 alike) : Display
  Forward Kinematics : WBToolboxLibrary/wholeBodyModel/Kinematics/Forward Kinematics  frameName=Frames.LEFT_FOOT
      settings: SourceProductName=Whole Body Toolbox
  Forward Kinematics1 : WBToolboxLibrary/wholeBodyModel/Kinematics/Forward Kinematics  frameName=Frames.RIGHT_FOOT
      settings: SourceProductName=Whole Body Toolbox
  MATLAB Function : MATLAB Function  TreatAsAtomicUnit=on
  w_H_humanLeftFeet : Outport
  w_H_humanRightFeet : Outport  Port=2
  wires:
  MATLAB Function/1(w_H_humanLeftFeet) -> w_H_humanLeftFeet/1
  Forward Kinematics1/1 -> Display4/1, MATLAB Function/2(w_H_robotRightFeet)
  Forward Kinematics/1 -> Display2/1, MATLAB Function/1(w_H_robotLeftFeet)
  qj/1 -> Display3/1, Forward Kinematics1/2, Forward Kinematics/2
  w_H_b/1 -> Display1/1, Forward Kinematics1/1, Forward Kinematics/1
  MATLAB Function/2(w_H_humanRightFeet) -> w_H_humanRightFeet/1

== system torqueBalancingPHRIStandup/Robot system/synchronizer ==
  GAZEBO_SYNCHRONIZER : Subsystem
  Logical Operator : Logic  Operator=NOT  AllPortsSameDT=off  OutDataTypeStr=boolean
  "ON_GAZEBO " : Constant  Value=Config.ON_GAZEBO
  REAL_TIME_SYNC : Subsystem
  To Workspace : ToWorkspace  VariableName=yarp_time  SaveFormat=Structure With Time  SampleTime=-1
  Yarp Clock : WBToolboxLibrary/Utilities/Yarp Clock
      settings: SourceProductName=Whole Body Toolbox
  wires:
  Logical Operator/1 -> REAL_TIME_SYNC/Enable
  "ON_GAZEBO "/1 -> GAZEBO_SYNCHRONIZER/Enable, Logical Operator/1
  Yarp Clock/1 -> To Workspace/1

== system torqueBalancingPHRIStandup/Assistant system/Real system/Contact Kinematics ==
  w_H_b : Inport
  qj : Inport  Port=2
  nu_b : Inport  Port=3
  qjdot : Inport  Port=4
  Arm Contact Kinematics : Subsystem
  Leg Contact Kinematics : Subsystem
  w_H_lFoot : Outport
  w_H_rFoot : Outport  Port=2
  JLFoot : Outport  Port=3
  JRFoot : Outport  Port=4
  dJLFootnu : Outport  Port=5
  dJRFootnu : Outport  Port=6
  w_H_lArm : Outport  Port=7
  w_H_rArm : Outport  Port=8
  JLArm : Outport  Port=9
  JRArm : Outport  Port=10
  dJLArmnu : Outport  Port=11
  dJRArmnu : Outport  Port=12
  wires:
  w_H_b/1 -> Arm Contact Kinematics/1(w_H_b), Leg Contact Kinematics/1(w_H_b)
  qj/1 -> Arm Contact Kinematics/2(qj), Leg Contact Kinematics/2(qj)
  nu_b/1 -> Leg Contact Kinematics/3(nu_b), Arm Contact Kinematics/3(nu_b)
  qjdot/1 -> Arm Contact Kinematics/4(qjdot), Leg Contact Kinematics/4(qjdot)
  Leg Contact Kinematics/1(w_H_lFoot) -> w_H_lFoot/1
  Leg Contact Kinematics/2(w_H_rFoot) -> w_H_rFoot/1
  Leg Contact Kinematics/3(JLFoot) -> JLFoot/1
  Leg Contact Kinematics/4(JRFoot) -> JRFoot/1
  Leg Contact Kinematics/5(dJLFootnu) -> dJLFootnu/1
  Leg Contact Kinematics/6(dJRFootnu) -> dJRFootnu/1
  Arm Contact Kinematics/2(w_H_rArm) -> w_H_rArm/1
  Arm Contact Kinematics/1(w_H_lArm) -> w_H_lArm/1
  Arm Contact Kinematics/3(JLArm) -> JLArm/1
  Arm Contact Kinematics/5(dJLArmnu) -> dJLArmnu/1
  Arm Contact Kinematics/6(dJRArmnu) -> dJRArmnu/1
  Arm Contact Kinematics/4(JRArm) -> JRArm/1

== system torqueBalancingPHRIStandup/Assistant system/Real system/Dump and visualize ==
  Assistant Data : Subsystem
  Logical Operator1 : Logic  Operator=OR  AllPortsSameDT=off  OutDataTypeStr=boolean
  ON_GAZEBO 3 : Constant  Value=Config.SCOPES_ALL
  ON_GAZEBO 4 : Constant  Value=Config.SCOPES_MAIN
  wires:
  ON_GAZEBO 3/1 -> Logical Operator1/1
  ON_GAZEBO 4/1 -> Logical Operator1/2
  Logical Operator1/1 -> Assistant Data/Enable
  [assistant_jointVelocitiesData] -> Assistant Data/3(assistant_jointVelocitiesData)
  [assistant_jointTorquesData] -> Assistant Data/4(assistant_jointTorquesData)
  [assistant_w_H_b] -> Assistant Data/1(assistant_w_H_b)
  [assistant_jointData] -> Assistant Data/2(assistant_jointData)

== system torqueBalancingPHRIStandup/Assistant system/Real system/Dynamics ==
  w_H_b : Inport
  qj : Inport  Port=2
  nu_b : Inport  Port=3
  qjdot : Inport  Port=4
  Get Bias Forces : WBToolboxLibrary/wholeBodyModel/Dynamics/Get Bias Forces
      settings: SourceProductName=Whole Body Toolbox
  Mass Matrix : WBToolboxLibrary/wholeBodyModel/Dynamics/Mass Matrix
      settings: SourceProductName=Whole Body Toolbox
  M : Outport
  h : Outport  Port=2
  wires:
  qjdot/1 -> Get Bias Forces/4
  nu_b/1 -> Get Bias Forces/3
  qj/1 -> Get Bias Forces/2, Mass Matrix/2
  Get Bias Forces/1 -> h/1
  w_H_b/1 -> Get Bias Forces/1, Mass Matrix/1
  Mass Matrix/1 -> M/1

== system torqueBalancingPHRIStandup/Assistant system/Real system/Robot Model Position Control ==
  state : Inport
  q : Inport  Port=2
  Enable : EnablePort
  Clock : Clock
  Constant : Constant  Value=2
  Demux1 : Demux  Outputs=ASSISTANT_Config.numOfJointsForEachControlboard
  Minimum Jerk Trajectory Generator1 : WBToolboxLibrary/Utilities/Minimum Jerk Trajectory Generator  externalSettlingTime=on  settlingTime=1  sampleTime=Config.Ts  resetOnSettlingTime=off  firstDerivatives=off  secondDerivatives=off  explicitInitialValue=off
      settings: SourceProductName=Whole Body Toolbox
  Set References : WBToolboxLibrary/wholeBodyActuators/Set References  controlType=Position Direct  refSpeed=2*(pi/180)  refAcceleration=1000000*(pi/180)
      settings: SourceProductName=Whole Body Toolbox
  getJointRef : MATLAB Function  TreatAsAtomicUnit=on
  joint references : Scope  NumInputPorts=6
  wires:
  getJointRef/1(joint_ref) -> Minimum Jerk Trajectory Generator1/1
  Constant/1 -> Minimum Jerk Trajectory Generator1/2
  Demux1/3 -> joint references/3  "right_arm"
  Demux1/5 -> joint references/5  "right_leg"
  Demux1/4 -> joint references/4  "left_leg"
  Demux1/2 -> joint references/2  "left_arm"
  Minimum Jerk Trajectory Generator1/1 -> Demux1/1, Set References/1
  state/1 -> getJointRef/3(state), joint references/6
  Demux1/1 -> joint references/1  "torso"
  Clock/1 -> getJointRef/1(sim_time)
  q/1 -> getJointRef/2(q)

== system torqueBalancingPHRIStandup/Assistant system/Real system/Subsystem ==
  robot_w_H_assistant_LeftFeet : Inport
  robot_w_H_assistant_RightFeet : Inport  Port=2
  qj : Inport  Port=3
  Constant3 : Constant  Value=eye(4)
  Forward Kinematics : WBToolboxLibrary/wholeBodyModel/Kinematics/Forward Kinematics  frameName=ASSISTANT_Frames.LEFT_FOOT
      settings: SourceProductName=Whole Body Toolbox
  "Inv\\*  " : Product  Inputs=*/  Multiplication=Matrix(*)
  Switch : Switch  Criteria=u2 > Threshold
  switch threshold : Constant
  robot_w_H_assistant_base : Outport
  wires:
  robot_w_H_assistant_RightFeet/1 -> Switch/3
  "Inv\\*  "/1 -> robot_w_H_assistant_base/1
  qj/1 -> Forward Kinematics/2
  switch threshold/1 -> Switch/2
  Constant3/1 -> Forward Kinematics/1
  Switch/1 -> "Inv\\*  "/1
  Forward Kinematics/1 -> "Inv\\*  "/2
  robot_w_H_assistant_LeftFeet/1 -> Switch/1

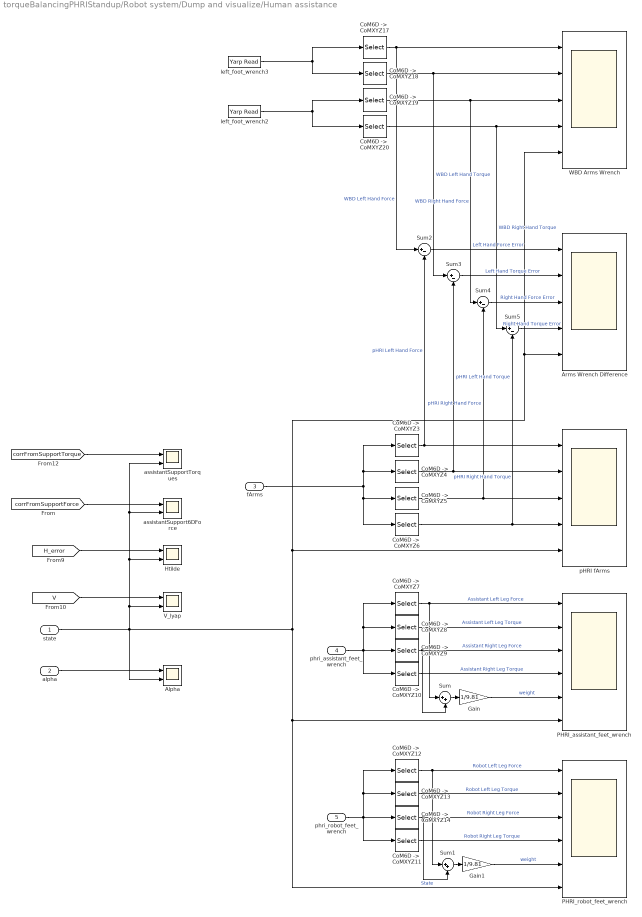
== system torqueBalancingPHRIStandup/Robot system/Dump and visualize/Human assistance ==
  state : Inport
  alpha : Inport  Port=2
  fArms : Inport  Port=3
  phri_assistant_feet_wrench : Inport  Port=4
  phri_robot_feet_wrench : Inport  Port=5
  Alpha : Scope  NumInputPorts=2
  Arms Wrench Difference : Scope  NumInputPorts=5
  "CoM6D ->  CoMXYZ10" : Selector  InputPortWidth=12  IndexOptions=Index vector (dialog)  Indices=[10 11 12]  OutputSizes=1
  "CoM6D ->  CoMXYZ11" : Selector  InputPortWidth=12  IndexOptions=Index vector (dialog)  Indices=[10 11 12]  OutputSizes=1
  "CoM6D ->  CoMXYZ12" : Selector  InputPortWidth=12  IndexOptions=Index vector (dialog)  Indices=[1 2 3]  OutputSizes=1
  "CoM6D ->  CoMXYZ13" : Selector  InputPortWidth=12  IndexOptions=Index vector (dialog)  Indices=[4 5 6]  OutputSizes=1
  "CoM6D ->  CoMXYZ14" : Selector  InputPortWidth=12  IndexOptions=Index vector (dialog)  Indices=[7 8 9]  OutputSizes=1
  "CoM6D ->  CoMXYZ17" : Selector  InputPortWidth=6  IndexOptions=Index vector (dialog)  Indices=[1 2 3]  OutputSizes=1
  "CoM6D ->  CoMXYZ18" : Selector  InputPortWidth=6  IndexOptions=Index vector (dialog)  Indices=[4 5 6]  OutputSizes=1
  "CoM6D ->  CoMXYZ19" : Selector  InputPortWidth=6  IndexOptions=Index vector (dialog)  Indices=[1 2 3]  OutputSizes=1
  "CoM6D ->  CoMXYZ20" : Selector  InputPortWidth=6  IndexOptions=Index vector (dialog)  Indices=[4 5 6]  OutputSizes=1
  "CoM6D ->  CoMXYZ3" : Selector  InputPortWidth=12  IndexOptions=Index vector (dialog)  Indices=[1 2 3]  OutputSizes=1
  "CoM6D ->  CoMXYZ4" : Selector  InputPortWidth=12  IndexOptions=Index vector (dialog)  Indices=[4 5 6]  OutputSizes=1
  "CoM6D ->  CoMXYZ5" : Selector  InputPortWidth=12  IndexOptions=Index vector (dialog)  Indices=[7 8 9]  OutputSizes=1
  "CoM6D ->  CoMXYZ6" : Selector  InputPortWidth=12  IndexOptions=Index vector (dialog)  Indices=[10 11 12]  OutputSizes=1
  "CoM6D ->  CoMXYZ7" : Selector  InputPortWidth=12  IndexOptions=Index vector (dialog)  Indices=[1 2 3]  OutputSizes=1
  "CoM6D ->  CoMXYZ8" : Selector  InputPortWidth=12  IndexOptions=Index vector (dialog)  Indices=[4 5 6]  OutputSizes=1
  "CoM6D ->  CoMXYZ9" : Selector  InputPortWidth=12  IndexOptions=Index vector (dialog)  Indices=[7 8 9]  OutputSizes=1
  Gain : Gain  Gain=1/9.81
  Gain1 : Gain  Gain=1/9.81
  Htilde : Scope  NumInputPorts=2
  PHRI_assistant_feet_wrench : Scope  NumInputPorts=6
  PHRI_robot_feet_wrench : Scope  NumInputPorts=6
  Sum : Sum  Inputs=|++
  Sum1 : Sum  Inputs=|++
  Sum{2..5} (4 alike) : Sum  Inputs=|+-
  V_lyap : Scope  NumInputPorts=2
  WBD Arms Wrench : Scope  NumInputPorts=5
  assistantSupport6DForce : Scope  NumInputPorts=2
  assistantSupportTorques : Scope  NumInputPorts=2
  left_foot_wrench2 : WBToolboxLibrary/Utilities/Yarp Read  portName=Ports.RIGHT_ARM  signalSize=6  timeout=0.5  blocking=off  timestamp=off  autoconnect=on  errorOnConnection=on
      settings: SourceProductName=Whole Body Toolbox
  left_foot_wrench3 : WBToolboxLibrary/Utilities/Yarp Read  portName=Ports.LEFT_ARM  signalSize=6  timeout=0.5  blocking=off  timestamp=off  autoconnect=on  errorOnConnection=on
      settings: SourceProductName=Whole Body Toolbox
  pHRI fArms : Scope  NumInputPorts=5
  wires:
  [H_error] -> Htilde/1
  [corrFromSupportForce] -> assistantSupport6DForce/1
  [V] -> V_lyap/1
  "CoM6D ->  CoMXYZ12"/1 -> Sum1/1, PHRI_robot_feet_wrench/1  "Robot Left Leg Force"
  alpha/1 -> Alpha/1
  "CoM6D ->  CoMXYZ11"/1 -> PHRI_robot_feet_wrench/4  "Robot Right Leg Torque"
  "CoM6D ->  CoMXYZ3"/1 -> pHRI fArms/1, Sum2/2  "pHRI Left Hand Force"
  "CoM6D ->  CoMXYZ4"/1 -> Sum3/2, pHRI fArms/2  "pHRI Left Hand Torque"
  "CoM6D ->  CoMXYZ14"/1 -> Sum1/2, PHRI_robot_feet_wrench/3  "Robot Right Leg Force"
  phri_robot_feet_wrench/1 -> "CoM6D ->  CoMXYZ11"/1, "CoM6D ->  CoMXYZ14"/1, "CoM6D ->  CoMXYZ12"/1, "CoM6D ->  CoMXYZ13"/1
  "CoM6D ->  CoMXYZ10"/1 -> PHRI_assistant_feet_wrench/4  "Assistant Right Leg Torque"
  "CoM6D ->  CoMXYZ7"/1 -> Sum/1, PHRI_assistant_feet_wrench/1  "Assistant Left Leg Force"
  phri_assistant_feet_wrench/1 -> "CoM6D ->  CoMXYZ10"/1, "CoM6D ->  CoMXYZ9"/1, "CoM6D ->  CoMXYZ8"/1, "CoM6D ->  CoMXYZ7"/1
  "CoM6D ->  CoMXYZ8"/1 -> PHRI_assistant_feet_wrench/2  "Assistant Left Leg Torque"
  "CoM6D ->  CoMXYZ9"/1 -> Sum/2, PHRI_assistant_feet_wrench/3  "Assistant Right Leg Force"
  "CoM6D ->  CoMXYZ6"/1 -> pHRI fArms/4, Sum5/2  "pHRI Right Hand Torque"
  "CoM6D ->  CoMXYZ5"/1 -> Sum4/2, pHRI fArms/3  "pHRI Right Hand Force"
  "CoM6D ->  CoMXYZ13"/1 -> PHRI_robot_feet_wrench/2  "Robot Left Leg Torque"
  Sum/1 -> Gain/1
  Gain/1 -> PHRI_assistant_feet_wrench/5  "weight"
  Gain1/1 -> PHRI_robot_feet_wrench/5  "weight"
  Sum1/1 -> Gain1/1
  state/1 -> Alpha/2, pHRI fArms/5, WBD Arms Wrench/5, Arms Wrench Difference/5, PHRI_robot_feet_wrench/6, PHRI_assistant_feet_wrench/6, V_lyap/2, Htilde/2, assistantSupportTorques/2, assistantSupport6DForce/2  "State"
  fArms/1 -> "CoM6D ->  CoMXYZ6"/1, "CoM6D ->  CoMXYZ5"/1, "CoM6D ->  CoMXYZ4"/1, "CoM6D ->  CoMXYZ3"/1
  Sum2/1 -> Arms Wrench Difference/1  "Left Hand Force Error"
  Sum3/1 -> Arms Wrench Difference/2  "Left Hand Torque Error"
  Sum4/1 -> Arms Wrench Difference/3  "Right Hand Force Error"
  Sum5/1 -> Arms Wrench Difference/4  "Right Hand Torque Error"
  "CoM6D ->  CoMXYZ18"/1 -> Sum3/1, WBD Arms Wrench/2  "WBD Left Hand Torque"
  "CoM6D ->  CoMXYZ17"/1 -> Sum2/1, WBD Arms Wrench/1  "WBD Left Hand Force"
  left_foot_wrench3/1 -> "CoM6D ->  CoMXYZ18"/1, "CoM6D ->  CoMXYZ17"/1
  "CoM6D ->  CoMXYZ19"/1 -> Sum4/1, WBD Arms Wrench/3  "WBD Right Hand Force"
  "CoM6D ->  CoMXYZ20"/1 -> WBD Arms Wrench/4, Sum5/1  "WBD Right Hand Torque"
  left_foot_wrench2/1 -> "CoM6D ->  CoMXYZ20"/1, "CoM6D ->  CoMXYZ19"/1
  [corrFromSupportTorque] -> assistantSupportTorques/1

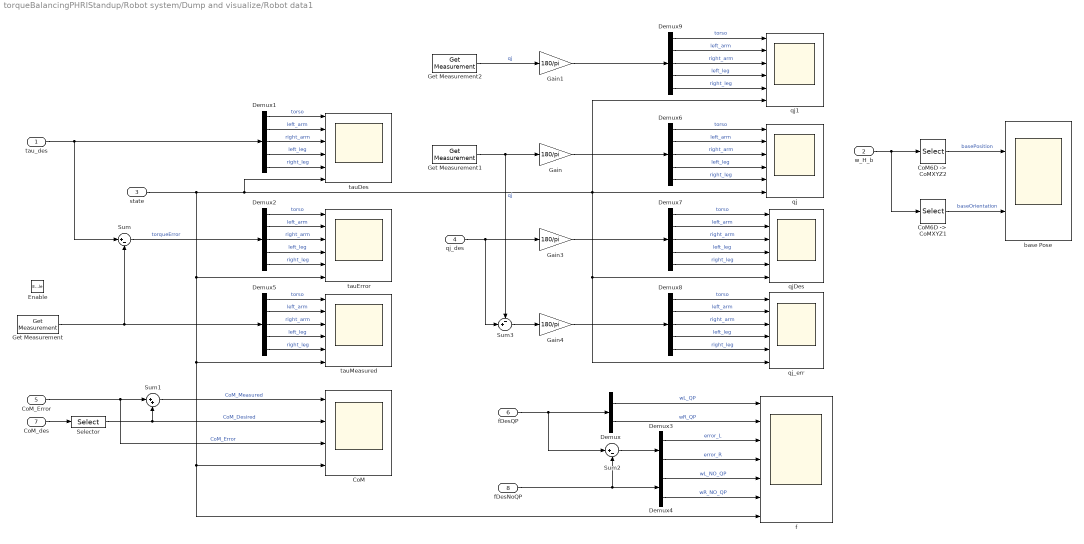
== system torqueBalancingPHRIStandup/Robot system/Dump and visualize/Robot data1 ==
  tau_des : Inport
  w_H_b : Inport  Port=2
  state : Inport  Port=3
  qj_des : Inport  Port=4
  CoM_Error : Inport  Port=5
  fDesQP : Inport  Port=6
  CoM_des : Inport  Port=7
  fDesNoQP : Inport  Port=8
  Enable : EnablePort
  CoM : Scope  NumInputPorts=4
  "CoM6D ->  CoMXYZ1" : Selector  NumberOfDimensions=2  InputPortWidth=7  IndexOptions=Index vector (dialog),Index vector (dialog)  Indices=[1 2 3],[1 2 3]  OutputSizes=1,1
  "CoM6D ->  CoMXYZ2" : Selector  NumberOfDimensions=2  InputPortWidth=7  IndexOptions=Index vector (dialog),Index vector (dialog)  Indices=[1 2 3],[4]  OutputSizes=1,1
  Demux : Demux  Outputs=2
  Demux{1..2,5..9} (7 alike) : Demux  Outputs=Config.numOfJointsForEachControlboard
  Demux3 : Demux  Outputs=2
  Demux4 : Demux  Outputs=2
  Gain{,1,3..4} (4 alike) : Gain  Gain=180/pi
  Get Measurement : WBToolboxLibrary/wholeBodyStates/Get Measurement  measuredType=Joints Torque
      settings: SourceProductName=Whole Body Toolbox
  Get Measurement1 : WBToolboxLibrary/wholeBodyStates/Get Measurement  measuredType=Joints Position
      settings: SourceProductName=Whole Body Toolbox
  Get Measurement2 : WBToolboxLibrary/wholeBodyStates/Get Measurement  measuredType=Joints Velocity
      settings: SourceProductName=Whole Body Toolbox
  Selector : Selector  NumberOfDimensions=2  IndexOptions=Index vector (dialog),Index vector (dialog)  Indices=[1:3],1  OutputSizes=1,1
  Sum : Sum  Inputs=|+-
  Sum1 : Sum  Inputs=|++
  Sum2 : Sum  Inputs=|+-
  Sum3 : Sum  Inputs=-+|
  base Pose : Scope  NumInputPorts=2
  f : Scope  NumInputPorts=7
  qj : Scope  NumInputPorts=6
  qj1 : Scope  NumInputPorts=6
  qjDes : Scope  NumInputPorts=6
  qj_err : Scope  NumInputPorts=6
  tauDes : Scope  NumInputPorts=6
  tauError : Scope  NumInputPorts=6
  tauMeasured : Scope  NumInputPorts=6
  wires:
  CoM_Error/1 -> Sum1/1, CoM/3  "CoM_Error"
  CoM_des/1 -> Selector/1
  Gain/1 -> Demux6/1
  Sum1/1 -> CoM/1  "CoM_Measured"
  Get Measurement1/1 -> Gain/1, Sum3/1  "qj"
  Demux6/5 -> qj/5  "right_leg"
  Demux6/1 -> qj/1  "torso"
  Demux6/2 -> qj/2  "left_arm"
  Demux6/4 -> qj/4  "left_leg"
  fDesQP/1 -> Sum2/1, Demux/1
  Demux6/3 -> qj/3  "right_arm"
  Sum2/1 -> Demux3/1
  fDesNoQP/1 -> Sum2/2, Demux4/1
  tau_des/1 -> Demux1/1, Sum/1
  Get Measurement/1 -> Demux5/1, Sum/2
  Demux1/5 -> tauDes/5  "right_leg"
  Demux1/1 -> tauDes/1  "torso"
  Demux1/2 -> tauDes/2  "left_arm"
  Demux1/4 -> tauDes/4  "left_leg"
  Demux1/3 -> tauDes/3  "right_arm"
  Demux2/5 -> tauError/5  "right_leg"
  Demux2/1 -> tauError/1  "torso"
  Demux2/2 -> tauError/2  "left_arm"
  Demux2/4 -> tauError/4  "left_leg"
  Demux2/3 -> tauError/3  "right_arm"
  Sum/1 -> Demux2/1  "torqueError"
  Demux5/5 -> tauMeasured/5  "right_leg"
  Demux5/1 -> tauMeasured/1  "torso"
  Demux5/2 -> tauMeasured/2  "left_arm"
  Demux5/4 -> tauMeasured/4  "left_leg"
  Demux5/3 -> tauMeasured/3  "right_arm"
  qj_des/1 -> Sum3/2, Gain3/1
  Gain3/1 -> Demux7/1
  Demux7/5 -> qjDes/5  "right_leg"
  Demux7/1 -> qjDes/1  "torso"
  Demux7/2 -> qjDes/2  "left_arm"
  Demux7/4 -> qjDes/4  "left_leg"
  Demux7/3 -> qjDes/3  "right_arm"
  Gain4/1 -> Demux8/1
  Demux8/5 -> qj_err/5  "right_leg"
  Demux8/1 -> qj_err/1  "torso"
  Demux8/2 -> qj_err/2  "left_arm"
  Demux8/4 -> qj_err/4  "left_leg"
  Demux8/3 -> qj_err/3  "right_arm"
  Sum3/1 -> Gain4/1
  Selector/1 -> Sum1/2, CoM/2  "CoM_Desired"
  Demux/1 -> f/1  "wL_QP"
  Demux/2 -> f/2  "wR_QP"
  Demux3/1 -> f/3  "error_L"
  Demux3/2 -> f/4  "error_R"
  Demux4/1 -> f/5  "wL_NO_QP"
  Demux4/2 -> f/6  "wR_NO_QP"
  w_H_b/1 -> "CoM6D ->  CoMXYZ1"/1, "CoM6D ->  CoMXYZ2"/1
  "CoM6D ->  CoMXYZ2"/1 -> base Pose/1  "basePosition"
  "CoM6D ->  CoMXYZ1"/1 -> base Pose/2  "baseOrientation"
  Demux9/5 -> qj1/5  "right_leg"
  Demux9/1 -> qj1/1  "torso"
  Demux9/2 -> qj1/2  "left_arm"
  Get Measurement2/1 -> Gain1/1  "qj"
  Demux9/4 -> qj1/4  "left_leg"
  Demux9/3 -> qj1/3  "right_arm"
  state/1 -> qj1/6, qj_err/6, qjDes/6, qj/6, tauDes/6, f/7, CoM/4, tauMeasured/6, tauError/6
  Gain1/1 -> Demux9/1
